simulink model "Simulaciones"  (R2022b)
settings: Solver=ode8  StartTime=0.0  StopTime=t6  FixedStep=0.01  RelTol=1e-3
values from neighbouring files (symbols this model uses):
  a0l = [0 0 0 cpL(1) 0 0; 0 0 0 0 cpL(2) 0; 0 0 0 0 0 cpL(3)]    [Superficies.m]
  alpha8 = -3    [Superficies.m]
  b = [1 0 0; 0 1 0; 0 0 1]    [Superficies.m]
  cL = [2;2;2]    [Superficies.m]
  cO = 2    [Superficies.m]
  cpL = [2;2;2]    [Superficies.m]
  cpO = 2    [Superficies.m]
  cpS = 0.2    [Superficies.m]
  cS = 0.2    [Superficies.m]
  gammaO = -3    [Superficies.m]
  gammaS = -2    [Superficies.m]
  k1 = 30    [Control.m]
  k2 = 1    [Control.m]
  k3 = 0.5    [Control.m]
  k4 = 0.001    [Control.m]
  klL = [1;1;1]    [Superficies.m]
  klO = 1    [Superficies.m]
  klS = 1    [Superficies.m]
  muO = 1    [Superficies.m]
  muS = 1    [Superficies.m]
  r8 = 1    [Superficies.m]
  t3 = tO + 1.0    (= 5.4)    [Trayectoria.m]
  xr8 = [xrxp; xryp; xrzp; 0; 0; 0]    [Trayectoria.m]
  xrLB = [xrxp; xryp; xrzp; 0; 0; 0]    [Trayectoria.m]
  xrLH = [xrxp; xryp; xrzp; 0; 0; 0]    [Trayectoria.m]
  xrLPA = [xrxp; xryp; xrzp; 0; 0; 0]    [Trayectoria.m]
  xrLR = [xrxp; xryp; xrzp; 0; 0; 0]    [Trayectoria.m]
  xrLSA = [xrxp; xryp; xrzp; 0; 0; 0]    [Trayectoria.m]
  xrLTA = [xrxp; xryp; xrzp; 0; 0; 0]    [Trayectoria.m]
  xrO = [xrxp; xryp; xrzp + sqrt(muO); 0; 0; 0]    [Trayectoria.m]
  xrS = [xrxp + sqrt(muS); xryp; xrzp; 0; 0; 0]    [Trayectoria.m]
undefined symbols (not defined in the file or in its folder): A, B, CI
libraries: vrlib x1
settings Model: Creator=olegalexandrocraviotog.  LastModifiedBy=olegalexandrocraviotog.

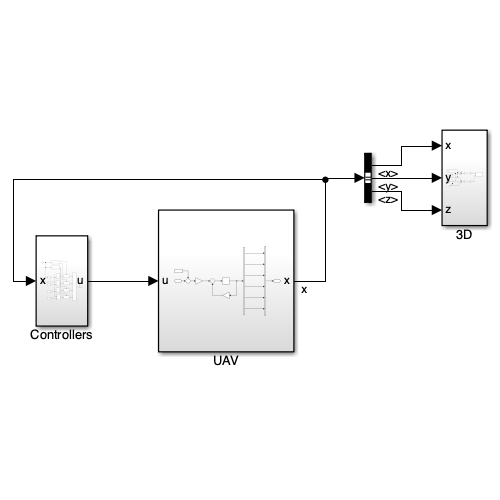
[thumbnail: Simulink's stored preview of the top-level diagram]
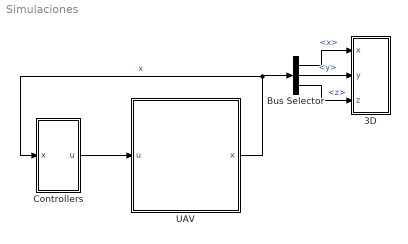
== system Simulaciones ==
  3D : Subsystem
  Bus Selector : BusSelector  OutputSignals=x,y,z
  Controllers : Subsystem
  UAV : Subsystem
  wires:
  Controllers/1(u) -> UAV/1(u)
  Bus Selector/3 -> 3D/3(z)  "<z>"
  Bus Selector/2 -> 3D/2(y)  "<y>"
  Bus Selector/1 -> 3D/1(x)  "<x>"
  UAV/1(x) -> Controllers/1(x), Bus Selector/1  "x"

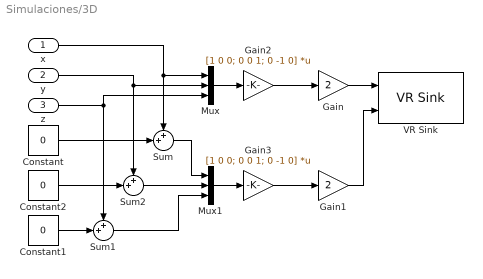
== system Simulaciones/3D ==
  x : Inport
  y : Inport  Port=2
  z : Inport  Port=3
  Constant : Constant  Value=0
  Constant1 : Constant  Value=0
  Constant2 : Constant  Value=0
  Gain : Gain  Gain=2
  Gain1 : Gain  Gain=2
  Gain2 : Gain  Gain=[1 0 0; 0 0 1; 0 -1 0]  Multiplication=Matrix(K*u)
  Gain3 : Gain  Gain=[1 0 0; 0 0 1; 0 -1 0]  Multiplication=Matrix(K*u)
  Mux : Mux  Inputs=3
  Mux1 : Mux  Inputs=3
  Sum : Sum  Inputs=++|
  Sum1 : Sum  Inputs=++|
  Sum2 : Sum  Inputs=++|
  VR Sink : vrlib/VR Sink  InstantiateOnLoad=on  SampleTime=0.01  ViewEnable=on  RemoteChange=off  RemoteView=off  FieldsWritten=Masa.translation.3.1.1.double#Pelota.position.3.1.1.double  WorldFileName=3D/Trayectoria3D.x3d  AutoView=off  VideoDimensions=[]  AllowVariableSize=off  FigureProperties="{'Position', 'Name', 'Viewpoint', 'CameraBound', 'CameraDirection', 'CameraPosition', 'CameraUpVector', 'ZoomFactor', 'Antialiasing', 'Headlight', 'Lighting', 'NavPanel', 'Sound', 'StatusBar', 'Stereo3D', 'Stereo3DCameraOffset', 'Stereo3DHIT', 'ToolBar', 'Textures', 'Transparency', 'Triad', 'Wireframe', 'NavZones', 'NavMode', 'NavSpeed', 'CaptureFileFormat', 'CaptureFileName', 'Record2DCompressMethod', 'Record2DCompressQuality', 'Record2D', 'Record2DFileName', 'Record2DFPS'; [2.2000000000000000e+01   1.0300000000000000e+02   5.7600000000000000e+02   3.5000000000000000e+02], '', 'Superior', 'on', [0.0000000000000000e+00   0.0000000000000000e+00  -1.0000000000000000e+00], [0.0000000000000000e+00   0.0000000000000000e+00   0.0000000000000000e+00], [0.0000000000000000e+00   1.0000000000000000e+00   0.0000000000000000e+00], [1.0000000000000000e+00], 'on', 'on', 'on', 'halfbar', 'on', 'on', 'off', [1.0000000149011612e-01], [0.0000000000000000e+00], 'on', 'on', 'on', 'none', 'off', 'off', 'fly', 'normal', 'tif', '%f_anim_%n.tif', 'auto', [7.5000000000000000e+01], 'on', '/Users/olegalexandrocraviotog./Downloads/%f_anim_%n.avi', 'auto'}"
  wires:
  z/1 -> Sum1/1, Mux/3
  y/1 -> Sum2/1, Mux/2
  x/1 -> Mux/1, Sum/1
  Gain2/1 -> Gain/1
  Mux/1 -> Gain2/1
  Sum1/1 -> Mux1/3
  Sum2/1 -> Mux1/2
  Sum/1 -> Mux1/1
  Gain3/1 -> Gain1/1
  Constant2/1 -> Sum2/2
  Constant1/1 -> Sum1/2
  Gain1/1 -> VR Sink/2
  Constant/1 -> Sum/2
  Mux1/1 -> Gain3/1
  Gain/1 -> VR Sink/1

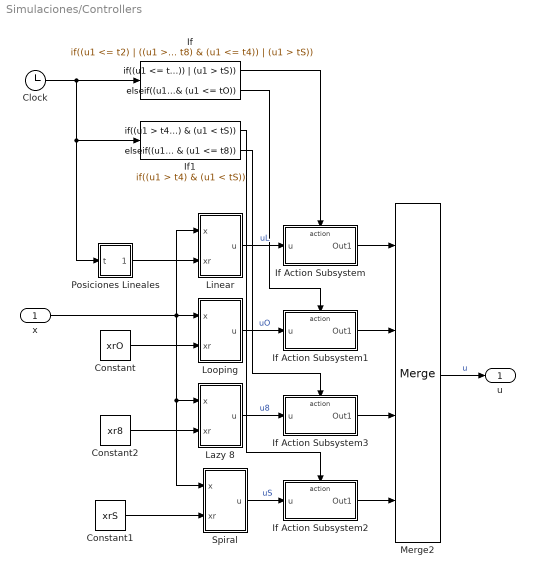
== system Simulaciones/Controllers ==
  x : Inport
  Clock : Clock
  Constant : Constant  Value=xrO
  Constant1 : Constant  Value=xrS
  Constant2 : Constant  Value=xr8
  If : If  IfExpression=(u1 <= t2) | ((u1 > tO) & (u1 <= t3)) | ((u1 > t8) & (u1 <= t4)) | (u1 > tS)  ElseIfExpressions=(u1 > t2) & (u1 <= tO)  ShowElse=off
  If Action Subsystem : Subsystem  TreatAsAtomicUnit=on
  If Action Subsystem1 : Subsystem  TreatAsAtomicUnit=on
  If Action Subsystem2 : Subsystem  TreatAsAtomicUnit=on
  If Action Subsystem3 : Subsystem  TreatAsAtomicUnit=on
  If1 : If  IfExpression=(u1 > t4) & (u1 < tS)  ElseIfExpressions=(u1 > t3) & (u1 <= t8)  ShowElse=off
  Lazy 8 : Subsystem
  Linear : Subsystem
  Looping : Subsystem
  Merge2 : Merge  Inputs=4
  Posiciones Lineales : Subsystem
  Spiral : Subsystem
  u : Outport
  wires:
  If1/1 -> If Action Subsystem2/Action
  If1/2 -> If Action Subsystem3/Action
  If/2 -> If Action Subsystem1/Action
  If/1 -> If Action Subsystem/Action
  Merge2/1 -> u/1  "u"
  Constant1/1 -> Spiral/2(xr)
  If Action Subsystem3/1(Out1) -> Merge2/3
  If Action Subsystem2/1(Out1) -> Merge2/4
  Posiciones Lineales/1(xr) -> Linear/2(xr)
  Clock/1 -> Posiciones Lineales/1(t), If1/1, If/1
  Constant2/1 -> Lazy 8/2(xr)
  Constant/1 -> Looping/2(xr)
  If Action Subsystem1/1(Out1) -> Merge2/2
  If Action Subsystem/1(Out1) -> Merge2/1
  Lazy 8/1(u) -> If Action Subsystem3/1(u)  "u8"
  Spiral/1(u) -> If Action Subsystem2/1(u)  "uS"
  Looping/1(u) -> If Action Subsystem1/1(u)  "uO"
  Linear/1(u) -> If Action Subsystem/1(u)  "uL"
  x/1 -> Looping/1(x), Linear/1(x), Lazy 8/1(x), Spiral/1(x)

== system Simulaciones/UAV ==
  u : Inport
  Bus Creator : BusCreator  Inputs=6
  Demux : Demux  Outputs=6
  Gain : Gain  Gain=A  Multiplication=Matrix(K*u)
  Gain1 : Gain  Gain=B  Multiplication=Matrix(K*u)
  Integrator : Integrator  InitialCondition=CI
  Perturbacion : Subsystem
  Sum : Sum  Inputs=|++
  Sum1 : Sum  Inputs=++|
  x : Outport
  wires:
  Perturbacion/1(xi) -> Sum1/1
  u/1 -> Sum1/2
  Sum1/1 -> Gain1/1
  Gain/1 -> Sum/2
  Gain1/1 -> Sum/1
  Integrator/1 -> Gain/1, Demux/1
  Bus Creator/1 -> x/1
  Demux/3 -> Bus Creator/3  "z"
  Demux/1 -> Bus Creator/1  "x"
  Sum/1 -> Integrator/1
  Demux/5 -> Bus Creator/5  "dy"
  Demux/2 -> Bus Creator/2  "y"
  Demux/6 -> Bus Creator/6  "dz"
  Demux/4 -> Bus Creator/4  "dx"

== system Simulaciones/Controllers/If Action Subsystem ==
  u : Inport
  Action Port : ActionPort  ActionPortLabel=if((u1 <= t2) | ((u1 > tO) & (u1 <= t3)) | ((u1 > t8) & (u1 <= t4)) | (u1 > tS))
  Out1 : Outport
  wires:
  u/1 -> Out1/1

== system Simulaciones/Controllers/If Action Subsystem1 ==
  u : Inport
  Action Port : ActionPort  ActionPortLabel=elseif((u1 > t2) & (u1 <= tO))
  Out1 : Outport
  wires:
  u/1 -> Out1/1

== system Simulaciones/Controllers/If Action Subsystem2 ==
  u : Inport
  Action Port : ActionPort  ActionPortLabel=if((u1 > t4) & (u1 < tS))
  Out1 : Outport
  wires:
  u/1 -> Out1/1

== system Simulaciones/Controllers/If Action Subsystem3 ==
  u : Inport
  Action Port : ActionPort  ActionPortLabel=elseif((u1 > t3) & (u1 <= t8))
  Out1 : Outport
  wires:
  u/1 -> Out1/1

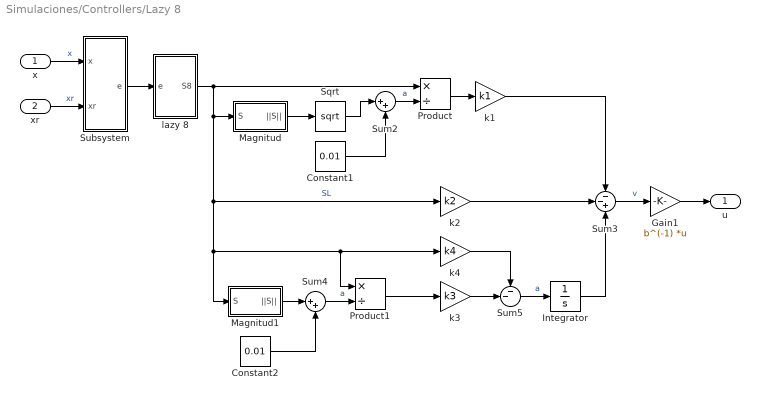
== system Simulaciones/Controllers/Lazy 8 ==
  x : Inport
  xr : Inport  Port=2
  Constant1 : Constant  Value=0.01
  Constant2 : Constant  Value=0.01
  Gain1 : Gain  Gain=b^(-1)  Multiplication=Matrix(K*u)
  Integrator : Integrator
  Magnitud : Subsystem
  Magnitud1 : Subsystem
  Product : Product  Inputs=*/
  Product1 : Product  Inputs=*/
  Sqrt : Sqrt
  Subsystem : Subsystem
  Sum2 : Sum  Inputs=|++
  Sum3 : Sum  Inputs=--+
  Sum4 : Sum  Inputs=|++
  Sum5 : Sum  Inputs=--|
  k1 : Gain  Gain=k1
  k2 : Gain  Gain=k2
  k3 : Gain  Gain=k3
  k4 : Gain  Gain=k4
  lazy 8 : Subsystem
  u : Outport
  wires:
  Sum3/1 -> Gain1/1  "v"
  xr/1 -> Subsystem/2(xr)  "xr"
  x/1 -> Subsystem/1(x)  "x"
  Subsystem/1(e) -> lazy 8/1(e)
  Gain1/1 -> u/1
  Integrator/1 -> Sum3/3
  Sum5/1 -> Integrator/1  "a"
  k4/1 -> Sum5/1
  k3/1 -> Sum5/2
  Product1/1 -> k3/1
  Magnitud1/1(||S||) -> Sum4/1
  Constant2/1 -> Sum4/2
  Sum4/1 -> Product1/2  "a"
  k2/1 -> Sum3/2
  k1/1 -> Sum3/1
  Sqrt/1 -> Sum2/1
  Magnitud/1(||S||) -> Sqrt/1
  Product/1 -> k1/1
  Constant1/1 -> Sum2/2
  Sum2/1 -> Product/2  "a"
  lazy 8/1(S8) -> Magnitud/1(S), Magnitud1/1(S), k4/1, Product1/1, k2/1, Product/1  "SL"

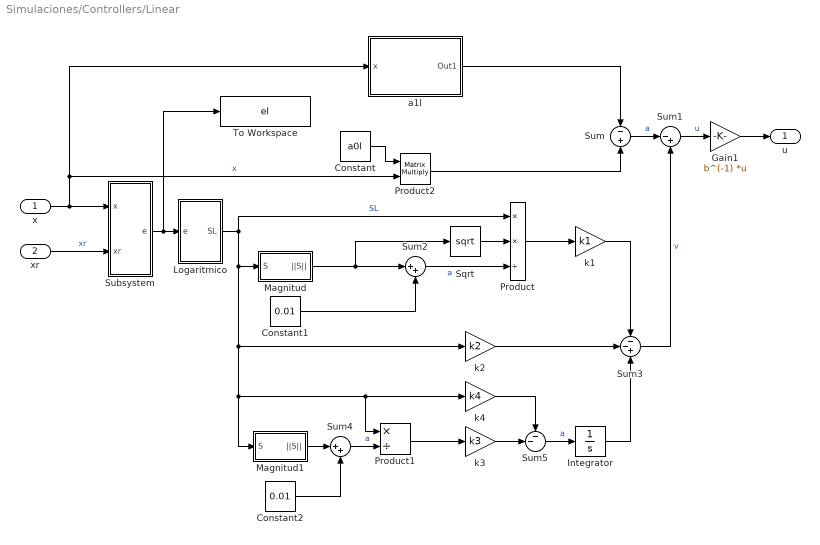
== system Simulaciones/Controllers/Linear ==
  x : Inport
  xr : Inport  Port=2
  Constant : Constant  Value=a0l
  Constant1 : Constant  Value=0.01
  Constant2 : Constant  Value=0.01
  Gain1 : Gain  Gain=b^(-1)  Multiplication=Matrix(K*u)
  Integrator : Integrator
  Logaritmico : Subsystem
  Magnitud : Subsystem
  Magnitud1 : Subsystem
  Product : Product  Inputs=**/
  Product1 : Product  Inputs=*/
  Product2 : Product  Inputs=**  Multiplication=Matrix(*)
  Sqrt : Sqrt
  Subsystem : Subsystem
  Sum : Sum  Inputs=-+
  Sum1 : Sum  Inputs=|-+
  Sum2 : Sum  Inputs=|++
  Sum3 : Sum  Inputs=--+
  Sum4 : Sum  Inputs=|++
  Sum5 : Sum  Inputs=--|
  To Workspace : ToWorkspace  VariableName=el  SampleTime=-1
  a1l : Subsystem
  k1 : Gain  Gain=k1
  k2 : Gain  Gain=k2
  k3 : Gain  Gain=k3
  k4 : Gain  Gain=k4
  u : Outport
  wires:
  a1l/1(Out1) -> Sum/1
  Product2/1 -> Sum/2
  Sum/1 -> Sum1/1  "a"
  Integrator/1 -> Sum3/3
  k2/1 -> Sum3/2
  Constant1/1 -> Sum2/2
  Sum2/1 -> Product/3  "a"
  Sqrt/1 -> Product/2
  xr/1 -> Subsystem/2(xr)  "xr"
  Subsystem/1(e) -> Logaritmico/1(e), To Workspace/1
  x/1 -> Product2/2, a1l/1(x), Subsystem/1(x)  "x"
  Logaritmico/1(SL) -> Product/1, k2/1, Product1/1, k4/1, Magnitud1/1(S), Magnitud/1(S)  "SL"
  Product/1 -> k1/1
  Magnitud/1(||S||) -> Sqrt/1, Sum2/1
  k1/1 -> Sum3/1
  Sum4/1 -> Product1/2  "a"
  Constant2/1 -> Sum4/2
  Magnitud1/1(||S||) -> Sum4/1
  Product1/1 -> k3/1
  k3/1 -> Sum5/2
  k4/1 -> Sum5/1
  Sum5/1 -> Integrator/1  "a"
  Sum1/1 -> Gain1/1  "u"
  Gain1/1 -> u/1
  Constant/1 -> Product2/1
  Sum3/1 -> Sum1/2  "v"

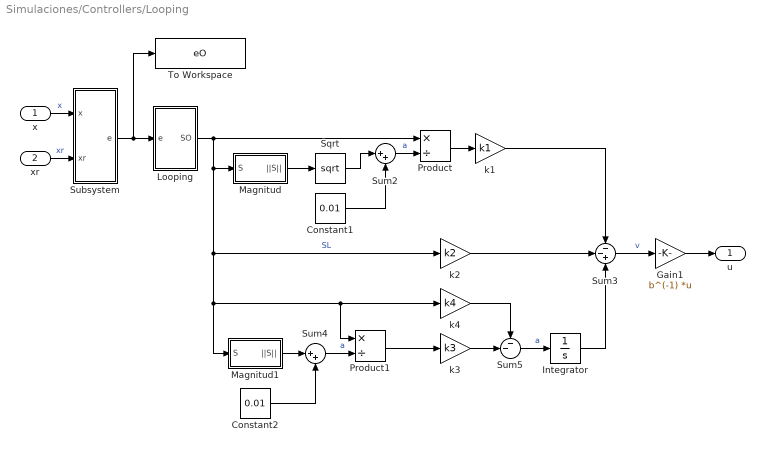
== system Simulaciones/Controllers/Looping ==
  x : Inport
  xr : Inport  Port=2
  Constant1 : Constant  Value=0.01
  Constant2 : Constant  Value=0.01
  Gain1 : Gain  Gain=b^(-1)  Multiplication=Matrix(K*u)
  Integrator : Integrator
  Looping : Subsystem
  Magnitud : Subsystem
  Magnitud1 : Subsystem
  Product : Product  Inputs=*/
  Product1 : Product  Inputs=*/
  Sqrt : Sqrt
  Subsystem : Subsystem
  Sum2 : Sum  Inputs=|++
  Sum3 : Sum  Inputs=--+
  Sum4 : Sum  Inputs=|++
  Sum5 : Sum  Inputs=--|
  To Workspace : ToWorkspace  VariableName=eO  SampleTime=-1
  k1 : Gain  Gain=k1
  k2 : Gain  Gain=k2
  k3 : Gain  Gain=k3
  k4 : Gain  Gain=k4
  u : Outport
  wires:
  Sum3/1 -> Gain1/1  "v"
  Subsystem/1(e) -> Looping/1(e), To Workspace/1
  xr/1 -> Subsystem/2(xr)  "xr"
  x/1 -> Subsystem/1(x)  "x"
  Gain1/1 -> u/1
  Integrator/1 -> Sum3/3
  Sum5/1 -> Integrator/1  "a"
  k4/1 -> Sum5/1
  k3/1 -> Sum5/2
  Product1/1 -> k3/1
  Magnitud1/1(||S||) -> Sum4/1
  Constant2/1 -> Sum4/2
  Sum4/1 -> Product1/2  "a"
  k2/1 -> Sum3/2
  k1/1 -> Sum3/1
  Sqrt/1 -> Sum2/1
  Magnitud/1(||S||) -> Sqrt/1
  Product/1 -> k1/1
  Constant1/1 -> Sum2/2
  Sum2/1 -> Product/2  "a"
  Looping/1(SO) -> Magnitud/1(S), Magnitud1/1(S), k4/1, Product1/1, k2/1, Product/1  "SL"

== system Simulaciones/Controllers/Posiciones Lineales ==
  t : Inport
  Finish : Subsystem  TreatAsAtomicUnit=on
  Hight : Subsystem  TreatAsAtomicUnit=on
  Hight finish : Subsystem  TreatAsAtomicUnit=on
  If : If  IfExpression=(u1 > tO) & (u1 <= t3)  ElseIfExpressions=(u1 > t8) & (u1 <= t4)  ShowElse=off
  If1 : If  IfExpression=u1 <= t1  ElseIfExpressions=(u1 > t1) & (u1 <= t2)  ShowElse=off
  If2 : If  IfExpression=(u1 > tS) & (u1 <= t5)  ElseIfExpressions=(u1 > t5)  ShowElse=off
  Lazy 8 position : Subsystem  TreatAsAtomicUnit=on
  Looping position : Subsystem  TreatAsAtomicUnit=on
  Merge2 : Merge  Inputs=6
  Spiral position : Subsystem  TreatAsAtomicUnit=on
  xr : Outport
  wires:
  If2/2 -> Finish/Action
  If2/1 -> Hight finish/Action
  If/2 -> Spiral position/Action
  If/1 -> Lazy 8 position/Action
  If1/2 -> Looping position/Action
  If1/1 -> Hight/Action
  t/1 -> If/1, If2/1, If1/1
  Finish/1(Out1) -> Merge2/6
  Hight finish/1(Out1) -> Merge2/5
  Spiral position/1(Out1) -> Merge2/4
  Lazy 8 position/1(Out1) -> Merge2/3
  Looping position/1(Out1) -> Merge2/2
  Hight/1(Out1) -> Merge2/1
  Merge2/1 -> xr/1  "UL"

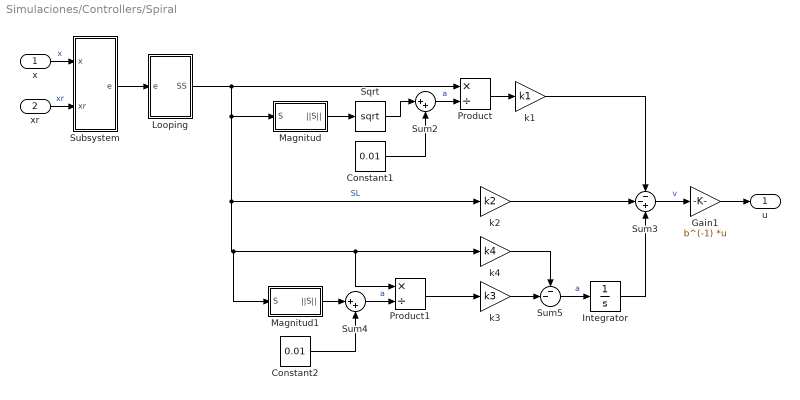
== system Simulaciones/Controllers/Spiral ==
  x : Inport
  xr : Inport  Port=2
  Constant1 : Constant  Value=0.01
  Constant2 : Constant  Value=0.01
  Gain1 : Gain  Gain=b^(-1)  Multiplication=Matrix(K*u)
  Integrator : Integrator
  Looping : Subsystem
  Magnitud : Subsystem
  Magnitud1 : Subsystem
  Product : Product  Inputs=*/
  Product1 : Product  Inputs=*/
  Sqrt : Sqrt
  Subsystem : Subsystem
  Sum2 : Sum  Inputs=|++
  Sum3 : Sum  Inputs=--+
  Sum4 : Sum  Inputs=|++
  Sum5 : Sum  Inputs=--|
  k1 : Gain  Gain=k1
  k2 : Gain  Gain=k2
  k3 : Gain  Gain=k3
  k4 : Gain  Gain=k4
  u : Outport
  wires:
  Looping/1(SS) -> Product/1, Magnitud/1(S), k2/1, k4/1, Product1/1, Magnitud1/1(S)  "SL"
  Subsystem/1(e) -> Looping/1(e)
  Sum3/1 -> Gain1/1  "v"
  xr/1 -> Subsystem/2(xr)  "xr"
  x/1 -> Subsystem/1(x)  "x"
  Sum2/1 -> Product/2  "a"
  Constant1/1 -> Sum2/2
  Product/1 -> k1/1
  Magnitud/1(||S||) -> Sqrt/1
  Sqrt/1 -> Sum2/1
  k1/1 -> Sum3/1
  k2/1 -> Sum3/2
  Sum4/1 -> Product1/2  "a"
  Constant2/1 -> Sum4/2
  Magnitud1/1(||S||) -> Sum4/1
  Product1/1 -> k3/1
  k3/1 -> Sum5/2
  k4/1 -> Sum5/1
  Sum5/1 -> Integrator/1  "a"
  Integrator/1 -> Sum3/3
  Gain1/1 -> u/1

== system Simulaciones/UAV/Perturbacion ==
  Clock : Clock
  Gain2 : Gain  Gain=0.35
  Gain3 : Gain  Gain=3.5
  Mux : Mux  Inputs=3
  Trigonometric Function : Trigonometry
  xi : Outport
  wires:
  Gain2/1 -> Mux/2, Mux/1, Mux/3
  Gain3/1 -> Trigonometric Function/1
  Mux/1 -> xi/1
  Clock/1 -> Gain3/1
  Trigonometric Function/1 -> Gain2/1

== system Simulaciones/Controllers/Lazy 8/Magnitud ==
  S : Inport
  Dot Product : DotProduct  OutDataTypeStr=Inherit: Inherit via internal rule
  Sqrt : Sqrt
  ||S|| : Outport
  wires:
  Dot Product/1 -> Sqrt/1
  S/1 -> Dot Product/1, Dot Product/2
  Sqrt/1 -> ||S||/1

== system Simulaciones/Controllers/Lazy 8/Magnitud1 ==
  S : Inport
  Dot Product : DotProduct  OutDataTypeStr=Inherit: Inherit via internal rule
  Sqrt : Sqrt
  ||S|| : Outport
  wires:
  Sqrt/1 -> ||S||/1
  S/1 -> Dot Product/2, Dot Product/1
  Dot Product/1 -> Sqrt/1

== system Simulaciones/Controllers/Lazy 8/Subsystem ==
  x : Inport
  xr : Inport  Port=2
  Bus Creator1 : BusCreator  Inputs=6
  Demux : Demux  Outputs=6
  Sum : Sum  Inputs=+-|
  e : Outport
  wires:
  Bus Creator1/1 -> e/1  "e"
  Sum/1 -> Demux/1  "e"
  x/1 -> Sum/1
  xr/1 -> Sum/2
  Demux/1 -> Bus Creator1/1  "ex"
  Demux/2 -> Bus Creator1/2  "ey"
  Demux/3 -> Bus Creator1/3  "ez"
  Demux/4 -> Bus Creator1/4  "dex"
  Demux/5 -> Bus Creator1/5  "dey"
  Demux/6 -> Bus Creator1/6  "dez"

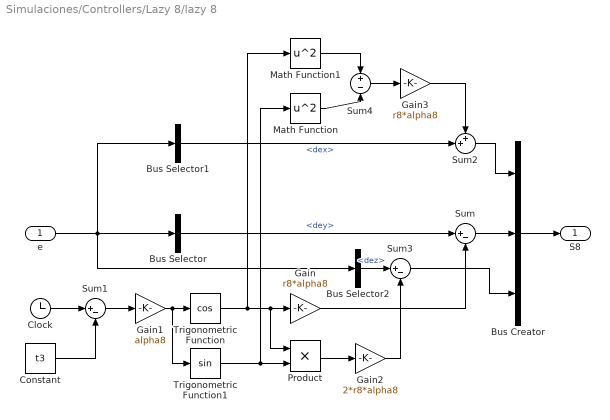
== system Simulaciones/Controllers/Lazy 8/lazy 8 ==
  e : Inport
  Bus Creator : BusCreator  Inputs=3
  Bus Selector : BusSelector  OutputSignals=dey
  Bus Selector1 : BusSelector  OutputSignals=dex
  Bus Selector2 : BusSelector  OutputSignals=dez
  Clock : Clock
  Constant : Constant  Value=t3
  Gain : Gain  Gain=r8*alpha8
  Gain1 : Gain  Gain=alpha8
  Gain2 : Gain  Gain=2*r8*alpha8
  Gain3 : Gain  Gain=r8*alpha8
  Math Function : Math  Operator=square
  Math Function1 : Math  Operator=square
  Product : Product
  Sum : Sum  Inputs=|+-
  Sum1 : Sum  Inputs=|+-
  Sum2 : Sum  Inputs=++|
  Sum3 : Sum  Inputs=|+-
  Sum4 : Sum  Inputs=+-
  Trigonometric Function : Trigonometry  Operator=cos
  Trigonometric Function1 : Trigonometry
  S8 : Outport
  wires:
  Sum4/1 -> Gain3/1
  Gain3/1 -> Sum2/1
  Math Function/1 -> Sum4/2
  Math Function1/1 -> Sum4/1
  Bus Selector1/1 -> Sum2/2  "<dex>"
  Sum3/1 -> Bus Creator/3
  Gain2/1 -> Sum3/2
  Bus Selector2/1 -> Sum3/1  "<dez>"
  Product/1 -> Gain2/1
  Trigonometric Function1/1 -> Product/2, Math Function/1
  Sum2/1 -> Bus Creator/1
  Constant/1 -> Sum1/2
  Sum1/1 -> Gain1/1
  Clock/1 -> Sum1/1
  Gain1/1 -> Trigonometric Function/1, Trigonometric Function1/1
  Gain/1 -> Sum/2
  Trigonometric Function/1 -> Product/1, Gain/1, Math Function1/1
  Sum/1 -> Bus Creator/2
  Bus Selector/1 -> Sum/1  "<dey>"
  e/1 -> Bus Selector/1, Bus Selector2/1, Bus Selector1/1
  Bus Creator/1 -> S8/1

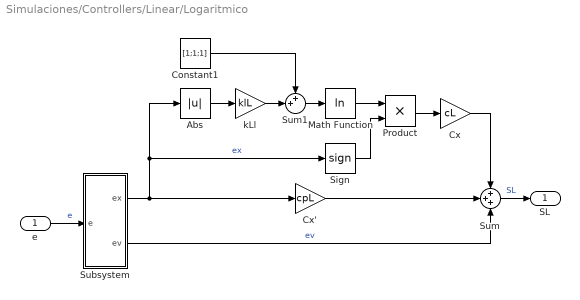
== system Simulaciones/Controllers/Linear/Logaritmico ==
  e : Inport
  Abs : Abs  SaturateOnIntegerOverflow=off
  Constant1 : Constant  Value=[1;1;1]
  Cx : Gain  Gain=cL
  Cx' : Gain  Gain=cpL
  Math Function : Math  Operator=log
  Product : Product
  Sign : Signum
  Subsystem : Subsystem
  Sum : Sum  Inputs=+++
  Sum1 : Sum  Inputs=++|
  kLl : Gain  Gain=klL
  SL : Outport
  wires:
  e/1 -> Subsystem/1(e)  "e"
  Subsystem/2(ev) -> Sum/3  "ev"
  Cx'/1 -> Sum/2
  Cx/1 -> Sum/1
  Subsystem/1(ex) -> Abs/1, Sign/1, Cx'/1  "ex"
  Sum/1 -> SL/1  "SL"
  Product/1 -> Cx/1
  Abs/1 -> kLl/1
  Constant1/1 -> Sum1/1
  Sum1/1 -> Math Function/1
  kLl/1 -> Sum1/2
  Sign/1 -> Product/2
  Math Function/1 -> Product/1

== system Simulaciones/Controllers/Linear/Magnitud ==
  S : Inport
  Dot Product : DotProduct  OutDataTypeStr=Inherit: Inherit via internal rule
  Sqrt : Sqrt
  ||S|| : Outport
  wires:
  Sqrt/1 -> ||S||/1
  S/1 -> Dot Product/2, Dot Product/1
  Dot Product/1 -> Sqrt/1

== system Simulaciones/Controllers/Linear/Magnitud1 ==
  S : Inport
  Dot Product : DotProduct  OutDataTypeStr=Inherit: Inherit via internal rule
  Sqrt : Sqrt
  ||S|| : Outport
  wires:
  Dot Product/1 -> Sqrt/1
  S/1 -> Dot Product/1, Dot Product/2
  Sqrt/1 -> ||S||/1

== system Simulaciones/Controllers/Linear/Subsystem ==
  x : Inport
  xr : Inport  Port=2
  Bus Creator1 : BusCreator  Inputs=6
  Demux : Demux  Outputs=6
  Sum : Sum  Inputs=+-|
  e : Outport
  wires:
  Bus Creator1/1 -> e/1  "e"
  Sum/1 -> Demux/1  "e"
  x/1 -> Sum/1
  xr/1 -> Sum/2
  Demux/1 -> Bus Creator1/1  "ex"
  Demux/2 -> Bus Creator1/2  "ey"
  Demux/3 -> Bus Creator1/3  "ez"
  Demux/4 -> Bus Creator1/4  "dex"
  Demux/5 -> Bus Creator1/5  "dey"
  Demux/6 -> Bus Creator1/6  "dez"

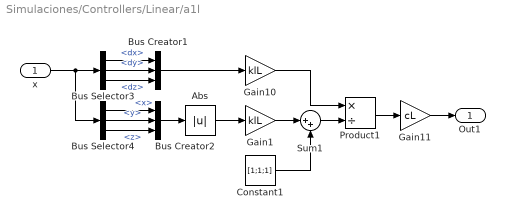
== system Simulaciones/Controllers/Linear/a1l ==
  x : Inport
  Abs : Abs  SaturateOnIntegerOverflow=off
  Bus Creator1 : BusCreator  Inputs=3
  Bus Creator2 : BusCreator  Inputs=3
  Bus Selector3 : BusSelector  OutputSignals=dx,dy,dz
  Bus Selector4 : BusSelector  OutputSignals=x,y,z
  Constant1 : Constant  Value=[1;1;1]
  Gain1 : Gain  Gain=klL
  Gain10 : Gain  Gain=klL
  Gain11 : Gain  Gain=cL
  Product1 : Product  Inputs=*/
  Sum1 : Sum  Inputs=|++
  Out1 : Outport
  wires:
  Abs/1 -> Gain1/1
  Product1/1 -> Gain11/1
  Sum1/1 -> Product1/2
  Gain11/1 -> Out1/1
  Bus Creator2/1 -> Abs/1
  Bus Creator1/1 -> Gain10/1
  Bus Selector4/1 -> Bus Creator2/1  "<x>"
  Bus Selector4/2 -> Bus Creator2/2  "<y>"
  Bus Selector4/3 -> Bus Creator2/3  "<z>"
  Bus Selector3/3 -> Bus Creator1/3  "<dz>"
  Bus Selector3/2 -> Bus Creator1/2  "<dy>"
  Bus Selector3/1 -> Bus Creator1/1  "<dx>"
  Constant1/1 -> Sum1/2
  Gain1/1 -> Sum1/1
  Gain10/1 -> Product1/1
  x/1 -> Bus Selector3/1, Bus Selector4/1

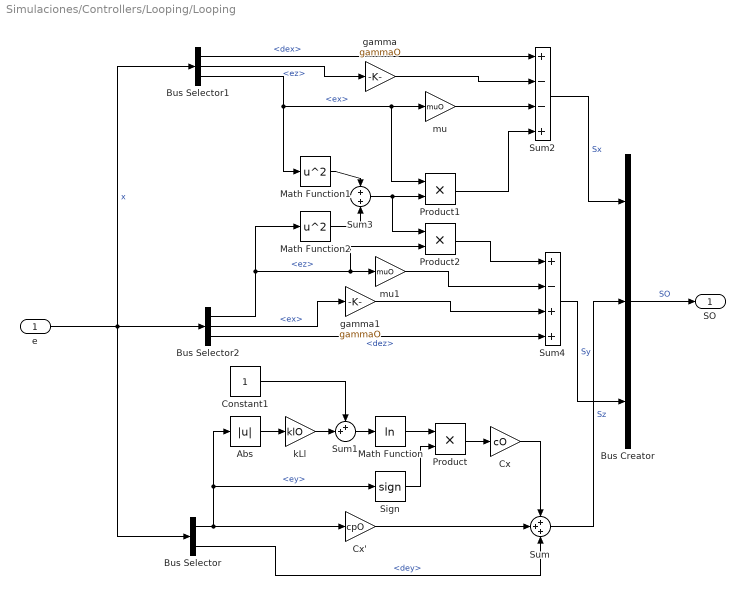
== system Simulaciones/Controllers/Looping/Looping ==
  e : Inport
  Abs : Abs  SaturateOnIntegerOverflow=off
  Bus Creator : BusCreator  Inputs=3
  Bus Selector : BusSelector  OutputSignals=ey,dey
  Bus Selector1 : BusSelector  OutputSignals=dex,ez,ex
  Bus Selector2 : BusSelector  OutputSignals=ez,ex,dez
  Constant1 : Constant
  Cx : Gain  Gain=cO
  Cx' : Gain  Gain=cpO
  Math Function : Math  Operator=log
  Math Function1 : Math  Operator=square
  Math Function2 : Math  Operator=square
  Product : Product
  Product1 : Product
  Product2 : Product
  Sign : Signum
  Sum : Sum  Inputs=+++
  Sum1 : Sum  Inputs=++|
  Sum2 : Sum  Inputs=+--+
  Sum3 : Sum
  Sum4 : Sum  Inputs=+-++
  gamma : Gain  Gain=gammaO
  gamma1 : Gain  Gain=gammaO
  kLl : Gain  Gain=klO
  mu : Gain  Gain=muO
  mu1 : Gain  Gain=muO
  SO : Outport
  wires:
  e/1 -> Bus Selector2/1, Bus Selector1/1, Bus Selector/1  "x"
  Sum2/1 -> Bus Creator/1  "Sx"
  Sum4/1 -> Bus Creator/3  "Sy"
  Bus Selector2/2 -> gamma1/1  "<ex>"
  Bus Selector2/3 -> Sum4/4  "<dez>"
  Bus Selector2/1 -> Math Function2/1, mu1/1, Product2/2  "<ez>"
  Bus Selector1/2 -> gamma/1  "<ez>"
  Bus Selector1/3 -> mu/1, Product1/1, Math Function1/1  "<ex>"
  Bus Selector1/1 -> Sum2/1  "<dex>"
  Sum/1 -> Bus Creator/2  "Sz"
  Bus Selector/2 -> Sum/3  "<dey>"
  Bus Selector/1 -> Abs/1, Sign/1, Cx'/1  "<ey>"
  Cx'/1 -> Sum/2
  Cx/1 -> Sum/1
  Product/1 -> Cx/1
  Abs/1 -> kLl/1
  Constant1/1 -> Sum1/1
  Sum1/1 -> Math Function/1
  kLl/1 -> Sum1/2
  Sign/1 -> Product/2
  Math Function/1 -> Product/1
  gamma/1 -> Sum2/2
  mu/1 -> Sum2/3
  Product1/1 -> Sum2/4
  Math Function2/1 -> Sum3/2
  Math Function1/1 -> Sum3/1
  Sum3/1 -> Product2/1, Product1/2
  Product2/1 -> Sum4/1
  gamma1/1 -> Sum4/3
  mu1/1 -> Sum4/2
  Bus Creator/1 -> SO/1  "SO"

== system Simulaciones/Controllers/Looping/Magnitud ==
  S : Inport
  Dot Product : DotProduct  OutDataTypeStr=Inherit: Inherit via internal rule
  Sqrt : Sqrt
  ||S|| : Outport
  wires:
  Dot Product/1 -> Sqrt/1
  S/1 -> Dot Product/1, Dot Product/2
  Sqrt/1 -> ||S||/1

== system Simulaciones/Controllers/Looping/Magnitud1 ==
  S : Inport
  Dot Product : DotProduct  OutDataTypeStr=Inherit: Inherit via internal rule
  Sqrt : Sqrt
  ||S|| : Outport
  wires:
  Sqrt/1 -> ||S||/1
  S/1 -> Dot Product/2, Dot Product/1
  Dot Product/1 -> Sqrt/1

== system Simulaciones/Controllers/Looping/Subsystem ==
  x : Inport
  xr : Inport  Port=2
  Bus Creator1 : BusCreator  Inputs=6
  Demux : Demux  Outputs=6
  Sum : Sum  Inputs=+-|
  e : Outport
  wires:
  Bus Creator1/1 -> e/1  "e"
  Sum/1 -> Demux/1  "e"
  x/1 -> Sum/1
  xr/1 -> Sum/2
  Demux/1 -> Bus Creator1/1  "ex"
  Demux/2 -> Bus Creator1/2  "ey"
  Demux/3 -> Bus Creator1/3  "ez"
  Demux/4 -> Bus Creator1/4  "dex"
  Demux/5 -> Bus Creator1/5  "dey"
  Demux/6 -> Bus Creator1/6  "dez"

== system Simulaciones/Controllers/Posiciones Lineales/Finish ==
  Action Port : ActionPort  ActionPortLabel=elseif((u1 > t5))
  Constant : Constant  Value=xrLB
  Out1 : Outport
  wires:
  Constant/1 -> Out1/1

== system Simulaciones/Controllers/Posiciones Lineales/Hight ==
  Action Port : ActionPort  ActionPortLabel=if(u1 <= t1)
  Constant : Constant  Value=xrLH
  Out1 : Outport
  wires:
  Constant/1 -> Out1/1

== system Simulaciones/Controllers/Posiciones Lineales/Hight finish ==
  Action Port : ActionPort  ActionPortLabel=if((u1 > tS) & (u1 <= t5))
  Constant : Constant  Value=xrLR
  Out1 : Outport
  wires:
  Constant/1 -> Out1/1

== system Simulaciones/Controllers/Posiciones Lineales/Lazy 8 position ==
  Action Port : ActionPort  ActionPortLabel=if((u1 > tO) & (u1 <= t3))
  Constant : Constant  Value=xrLSA
  Out1 : Outport
  wires:
  Constant/1 -> Out1/1

== system Simulaciones/Controllers/Posiciones Lineales/Looping position ==
  Action Port : ActionPort  ActionPortLabel=elseif((u1 > t1) & (u1 <= t2))
  Constant : Constant  Value=xrLPA
  Out1 : Outport
  wires:
  Constant/1 -> Out1/1

== system Simulaciones/Controllers/Posiciones Lineales/Spiral position ==
  Action Port : ActionPort  ActionPortLabel=elseif((u1 > t8) & (u1 <= t4))
  Constant : Constant  Value=xrLTA
  Out1 : Outport
  wires:
  Constant/1 -> Out1/1

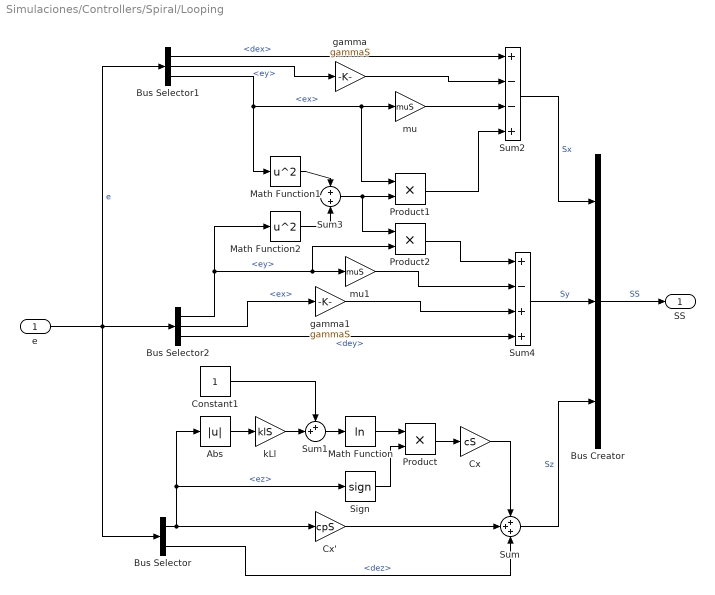
== system Simulaciones/Controllers/Spiral/Looping ==
  e : Inport
  Abs : Abs  SaturateOnIntegerOverflow=off
  Bus Creator : BusCreator  Inputs=3
  Bus Selector : BusSelector  OutputSignals=ez,dez
  Bus Selector1 : BusSelector  OutputSignals=dex,ey,ex
  Bus Selector2 : BusSelector  OutputSignals=ey,ex,dey
  Constant1 : Constant
  Cx : Gain  Gain=cS
  Cx' : Gain  Gain=cpS
  Math Function : Math  Operator=log
  Math Function1 : Math  Operator=square
  Math Function2 : Math  Operator=square
  Product : Product
  Product1 : Product
  Product2 : Product
  Sign : Signum
  Sum : Sum  Inputs=+++
  Sum1 : Sum  Inputs=++|
  Sum2 : Sum  Inputs=+--+
  Sum3 : Sum
  Sum4 : Sum  Inputs=+-++
  gamma : Gain  Gain=gammaS
  gamma1 : Gain  Gain=gammaS
  kLl : Gain  Gain=klS
  mu : Gain  Gain=muS
  mu1 : Gain  Gain=muS
  SS : Outport
  wires:
  e/1 -> Bus Selector2/1, Bus Selector1/1, Bus Selector/1  "e"
  Sum/1 -> Bus Creator/3  "Sz"
  Sum4/1 -> Bus Creator/2  "Sy"
  Bus Selector/2 -> Sum/3  "<dez>"
  Bus Selector/1 -> Cx'/1, Abs/1, Sign/1  "<ez>"
  Bus Selector2/3 -> Sum4/4  "<dey>"
  Bus Selector2/1 -> mu1/1, Product2/2, Math Function2/1  "<ey>"
  Bus Selector2/2 -> gamma1/1  "<ex>"
  Bus Selector1/2 -> gamma/1  "<ey>"
  Bus Creator/1 -> SS/1  "SS"
  mu1/1 -> Sum4/2
  gamma1/1 -> Sum4/3
  Product2/1 -> Sum4/1
  Sum3/1 -> Product1/2, Product2/1
  Math Function1/1 -> Sum3/1
  Math Function2/1 -> Sum3/2
  Product1/1 -> Sum2/4
  mu/1 -> Sum2/3
  gamma/1 -> Sum2/2
  Math Function/1 -> Product/1
  Sign/1 -> Product/2
  kLl/1 -> Sum1/2
  Sum1/1 -> Math Function/1
  Constant1/1 -> Sum1/1
  Abs/1 -> kLl/1
  Product/1 -> Cx/1
  Cx/1 -> Sum/1
  Cx'/1 -> Sum/2
  Bus Selector1/1 -> Sum2/1  "<dex>"
  Bus Selector1/3 -> Math Function1/1, Product1/1, mu/1  "<ex>"
  Sum2/1 -> Bus Creator/1  "Sx"

== system Simulaciones/Controllers/Spiral/Magnitud ==
  S : Inport
  Dot Product : DotProduct  OutDataTypeStr=Inherit: Inherit via internal rule
  Sqrt : Sqrt
  ||S|| : Outport
  wires:
  Sqrt/1 -> ||S||/1
  S/1 -> Dot Product/2, Dot Product/1
  Dot Product/1 -> Sqrt/1

== system Simulaciones/Controllers/Spiral/Magnitud1 ==
  S : Inport
  Dot Product : DotProduct  OutDataTypeStr=Inherit: Inherit via internal rule
  Sqrt : Sqrt
  ||S|| : Outport
  wires:
  Dot Product/1 -> Sqrt/1
  S/1 -> Dot Product/1, Dot Product/2
  Sqrt/1 -> ||S||/1

== system Simulaciones/Controllers/Spiral/Subsystem ==
  x : Inport
  xr : Inport  Port=2
  Bus Creator1 : BusCreator  Inputs=6
  Demux : Demux  Outputs=6
  Sum : Sum  Inputs=+-|
  e : Outport
  wires:
  Bus Creator1/1 -> e/1  "e"
  Sum/1 -> Demux/1  "e"
  x/1 -> Sum/1
  xr/1 -> Sum/2
  Demux/1 -> Bus Creator1/1  "ex"
  Demux/2 -> Bus Creator1/2  "ey"
  Demux/3 -> Bus Creator1/3  "ez"
  Demux/4 -> Bus Creator1/4  "dex"
  Demux/5 -> Bus Creator1/5  "dey"
  Demux/6 -> Bus Creator1/6  "dez"

== system Simulaciones/Controllers/Linear/Logaritmico/Subsystem ==
  e : Inport
  Bus Creator : BusCreator  Inputs=3
  Bus Creator1 : BusCreator  Inputs=3
  Demux : Demux  Outputs=6
  ex : Outport
  ev : Outport  Port=2
  wires:
  e/1 -> Demux/1
  Bus Creator1/1 -> ev/1
  Demux/6 -> Bus Creator1/3  "dez"
  Demux/5 -> Bus Creator1/2  "dey"
  Demux/4 -> Bus Creator1/1  "dex"
  Bus Creator/1 -> ex/1
  Demux/3 -> Bus Creator/3  "ez"
  Demux/2 -> Bus Creator/2  "ey"
  Demux/1 -> Bus Creator/1  "ex"
